simulink model "commtailbiting"  (R2023b)
settings: Solver=FixedStepDiscrete  StartTime=0.0  StopTime=3600  RelTol=1e-3
PreLoadFcn:
  | blkLen = 100;
  | EbNo = 4;
  | maxNumErrs = 1000;
  | maxNumBits = 5e6;
libraries: commcnvcod2 x3, commdigbbndpm3 x2, commchan3 x1, commrandsrc3 x1, commsink2 x1
Description:
  | Tail-biting convolutional coding example model
settings Model: Creator=The MathWorks, Inc.  LastModifiedBy=yuvra
settings SolverCC: AlgebraicLoopSolver=TrustRegion
settings DataIOCC: LimitDataPoints=on  SaveFormat=Array  ReturnWorkspaceOutputs=off
settings OptimizationCC: ReuseModelBlockBuffer=off  ExpressionDepthLimit=2147483647  InitFltsAndDblsToZero=on  EfficientMapNaN2IntZero=off  LifeSpan=inf
settings DebuggingCC: SolverPrmCheckMsg=warning  UnconnectedInputMsg=warning  UnconnectedOutputMsg=warning  UnconnectedLineMsg=warning  AllowSymbolicDim=off  StateNameClashWarn=warning  SFUnexpectedBacktrackingDiag=warning  SFNoUnconditionalDefaultTransitionDiag=warning  SFExecutionAtInitializationDiag=none  ArithmeticOperatorsInVariantConditions=warning
settings HardwareCC: ProdBitPerPointer=32  ProdBitPerSizeT=32  ProdBitPerPtrDiffT=32  ProdLargestAtomicFloat=None  ProdIntDivRoundTo=Undefined  ProdEndianess=Unspecified  ProdWordSize=32  ProdHWDeviceType=32-bit Generic
settings ModelReferenceCC: EnableRefExpFcnMdlSchedulingChecks=on  PropagateSignalLabelsOutOfModel=off
settings SFSimCC: SimUseLocalCustomCode=off  CustomCodeUndefinedFunction=UseInterfaceOnly
settings RTWCC: RTWUseLocalCustomCode=off
settings CodeAppCC: StateflowObjectComments=on
settings GRTTargetCC: TargetLangStandard=C89/C90 (ANSI)  CombineOutputUpdateFcns=off  GRTInterface=on
settings ConfigComp: CovMetricSettings=dw  CovSaveCumulativeToWorkspaceVar=on  CovSaveSingleToWorkspaceVar=on  CovExternalEMLEnable=off  CovSFcnEnable=off

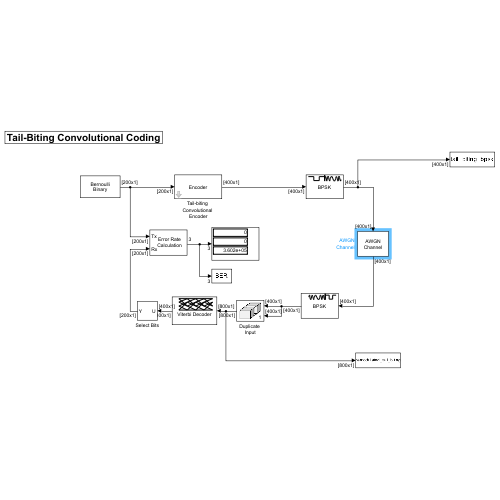
[thumbnail: Simulink's stored preview of the top-level diagram]
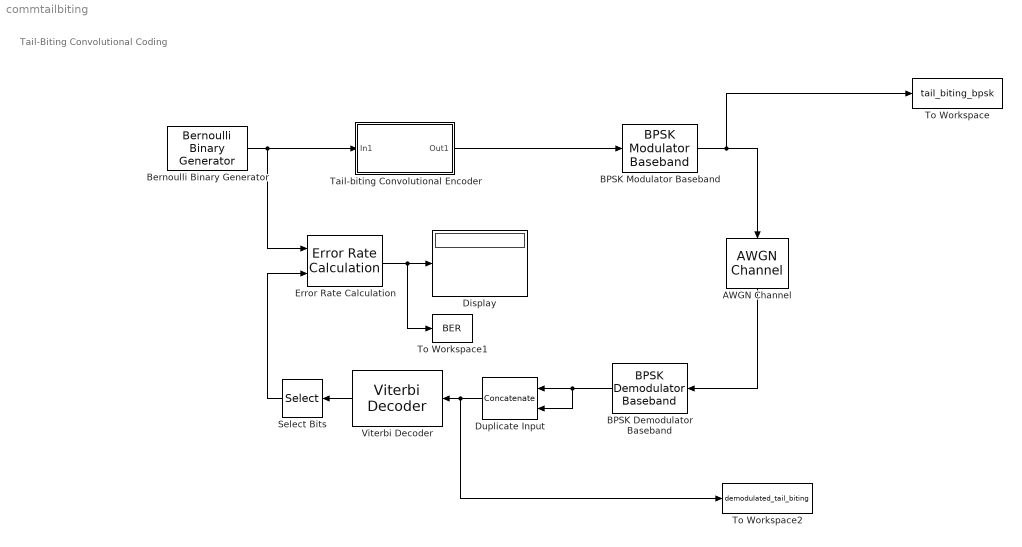
== system commtailbiting ==
  note: Tail-Biting Convolutional Coding
  AWGN Channel : commchan3/AWGN Channel  LegacyMode=off  NoiseMethod="Signal to noise ratio  (SNR)"  noiseMode="Signal to noise ratio  (Eb/No)"  EbNo=0  EsNo=EbNo + 10*log10(1/2)  SNR=10  BitsPerSymbol=1  SignalPower=1  SamplesPerSymbol=2  SymbolPeriod=0.01  VarianceSource=Parameter  Variance=1  RandomStream=mt19937ar with seed  Seed=67  SimulateUsing=Interpreted execution
  BPSK Demodulator Baseband : commdigbbndpm3/BPSK Demodulator Baseband  DecType=Hard decision  VarSource=Dialog  Variance=1  Ph=0  outDtype=boolean  derotateFactorWordLen=16  derotateFactorDataTypeStr=Inherit: Same word length as input  derotateFactorLastDataTypeStr=Inherit: Same word length as input
  BPSK Modulator Baseband : commdigbbndpm3/BPSK Modulator Baseband  Ph=0  outDtype=double  outWordLen=16  outUDDataType=sfix(16)  outFracLenMode=Best precision  outFracLen=15  outDataTypeStr=double  outLastDataTypeStr=double
  Bernoulli Binary Generator : commrandsrc3/Bernoulli Binary Generator  ProbabilityOfZero=0.5  SeedSource=Parameter  Seed=61  SampleTime=0.01  SamplesPerFrame=blkLen  OutputDataType=boolean  SimulateUsing=Interpreted execution
  Display : Display
  Duplicate Input : Concatenate  Mode=Multidimensional array
  Error Rate Calculation : commsink2/Error Rate Calculation  N=0  st_delay=0  cp_mode=Entire frame  subframe=[]  PMode=Port  WsName=ErrorVec  RsMode2=off  stop=on  numErr=maxNumErrs  maxBits=maxNumBits
  Select Bits : Selector  NumberOfDimensions=2  InputPortWidth=3  IndexOptions=Index vector (dialog),Select all  Indices=[blkLen+1:(3*blkLen/2) (blkLen/2+1):blkLen],1  OutputSizes=1,1
  Tail-biting Convolutional Encoder : Subsystem  mask(Tail-Biting Convolutional Encoder){trellis=poly2trellis(7, [171 133])}
      mask prompts: trellis "Trellis structure:"
      mask init:
      | mLen = log2(trellis.numStates);
      mask Display: disp('Encoder');
  To Workspace : ToWorkspace  VariableName=tail_biting_bpsk  SampleTime=-1
  To Workspace1 : ToWorkspace  VariableName=BER  SampleTime=-1
      settings: MaxDataPoints=1
  To Workspace2 : ToWorkspace  VariableName=demodulated_tail_biting  SampleTime=-1
  Viterbi Decoder : commcnvcod2/Viterbi Decoder  trellis=poly2trellis(7, [171 133])  isPunctured=off  punctureVector=[1; 1; 0; 1; 0; 1]  erasures=off  dectype=Hard decision  nsdecb=4  runSigValErrCheck=off  tbdepth=34  opmode=Truncated  reset=off  delayedResetAction=off  smWordLength=16  outDataType=boolean
  wires:
  Bernoulli Binary Generator/1 -> Tail-biting Convolutional Encoder/1(In1), Error Rate Calculation/1
  Tail-biting Convolutional Encoder/1(Out1) -> BPSK Modulator Baseband/1
  Duplicate Input/1 -> To Workspace2/1, Viterbi Decoder/1
  Viterbi Decoder/1 -> Select Bits/1
  Select Bits/1 -> Error Rate Calculation/2
  BPSK Demodulator Baseband/1 -> Duplicate Input/1, Duplicate Input/2
  AWGN Channel/1 -> BPSK Demodulator Baseband/1
  BPSK Modulator Baseband/1 -> To Workspace/1, AWGN Channel/1
  Error Rate Calculation/1 -> Display/1, To Workspace1/1

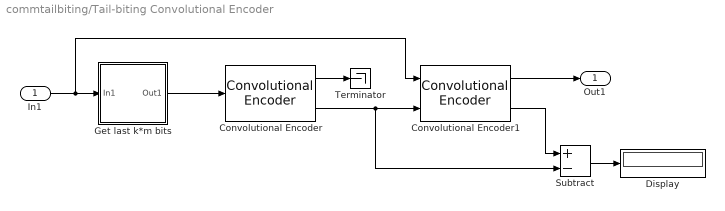
== system commtailbiting/Tail-biting Convolutional Encoder ==
  In1 : Inport
  Convolutional Encoder : commcnvcod2/Convolutional Encoder  trellis=trellis  opMode=Truncated (reset every frame)  DelayedResetAction=off  hasIniStPort=off  hasFinStPort=on  usePuncVector=off  punctureVector=[1; 1; 0; 1; 0; 1]  reset=Unused parameter value
  Convolutional Encoder1 : commcnvcod2/Convolutional Encoder  trellis=trellis  opMode=Truncated (reset every frame)  DelayedResetAction=off  hasIniStPort=on  hasFinStPort=on  usePuncVector=off  punctureVector=[1; 1; 0; 1; 0; 1]  reset=Unused parameter value
  Display : Display
  Get last k*m bits : Subsystem  mask{m=mLen}
      mask prompts: m "Memory length:"
      mask Display: disp('Extract bits')
  Subtract : Sum  Inputs=+-
  Terminator : Terminator
  Out1 : Outport  VectorParamsAs1DForOutWhenUnconnected=off
  wires:
  In1/1 -> Get last k*m bits/1(In1), Convolutional Encoder1/1
  Get last k*m bits/1(Out1) -> Convolutional Encoder/1
  Convolutional Encoder/2 -> Convolutional Encoder1/2, Subtract/2
  Convolutional Encoder1/1 -> Out1/1
  Convolutional Encoder/1 -> Terminator/1
  Convolutional Encoder1/2 -> Subtract/1
  Subtract/1 -> Display/1

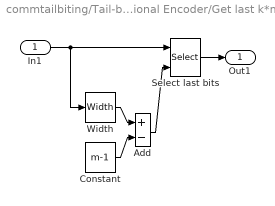
== system commtailbiting/Tail-biting Convolutional Encoder/Get last k*m bits ==
  In1 : Inport
  Add : Sum  Inputs=+-
  Constant : Constant  Value=m-1
  Select last bits : Selector  NumberOfDimensions=2  InputPortWidth=3  IndexOptions=Starting index (port),Select all  Indices=32-6:32,1  OutputSizes=m,1
  Width : Width
  Out1 : Outport  VectorParamsAs1DForOutWhenUnconnected=off
  wires:
  In1/1 -> Select last bits/1, Width/1
  Width/1 -> Add/1
  Constant/1 -> Add/2
  Add/1 -> Select last bits/2
  Select last bits/1 -> Out1/1
